simulink model "PSK"  (R2020a)
settings: Solver=FixedStepAuto  StartTime=0.0  StopTime=10.0  FixedStep=0.01  RelTol=1e-3
settings Model: Creator=AVS  LastModifiedBy=AVS

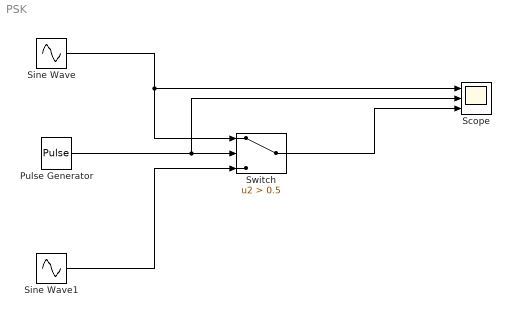
== system PSK ==
  Pulse Generator : DiscretePulseGenerator  PulseType=Time based  PulseWidth=50
  Scope : Scope  NumInputPorts=3
  Sine Wave : Sin  Frequency=2*pi*2  SampleTime=0.01
  Sine Wave1 : Sin  Frequency=2*pi*2  Phase=pi  SampleTime=0.01
  Switch : Switch  Criteria=u2 > Threshold  Threshold=0.5
  wires:
  Pulse Generator/1 -> Scope/2, Switch/2
  Sine Wave1/1 -> Switch/3
  Sine Wave/1 -> Switch/1, Scope/1
  Switch/1 -> Scope/3
